simulink model "MVB3single"  (R2013b)
settings: Solver=FixedStepDiscrete  SolverMode=SingleTasking  StartTime=0  StopTime=5000  RelTol=1e-3
model workspace (MAT data in the model file):
  logicAddr = 2
settings Model: Creator=qiji  LastModifiedBy=qiji
settings DataIOCC: SignalLoggingSaveFormat=ModelDataLogs
settings OptimizationCC: BlockReduction=off  ConditionallyExecuteInputs=off  InlineParams=on
settings DebuggingCC: UnderspecifiedInitializationDetection=Simplified  MultiTaskDSMMsg=warning  MultiTaskCondExecSysMsg=none  SingleTaskRateTransMsg=error  SFUnusedDataAndEventsDiag=none
settings RTWCC: IncludeERTFirstTime=on
settings GRTTargetCC: CodeReplacementLibrary=None  CPPClassGenCompliant=on
settings ConfigurationSet: Description=SimMechanics 2G

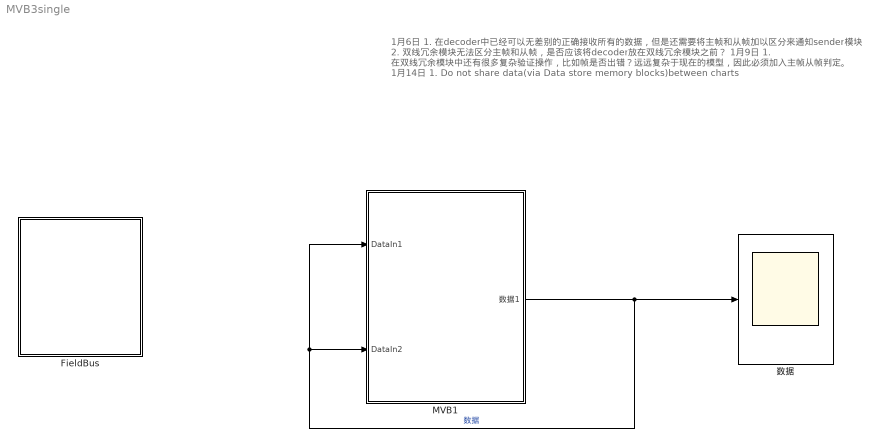
== system MVB3single ==
  note: 1月6日
      | 1. 在decoder中已经可以无差别的正确接收所有的数据，但是还需要将主帧和从帧加以区分来通知sender模块
      | 2. 双线冗余模块无法区分主帧和从帧，是否应该将decoder放在双线冗余模块之前？
      | 1月9日
      | 1. 在双线冗余模块中还有很多复杂验证操作，比如帧是否出错？远远复杂于现在的模型，因此必须加入主帧从帧判定。
      | 1月14日
      | 1. Do not share data(via Data store memory blocks)between charts
  FieldBus : Subsystem
  MVB1 : Subsystem
  数据 : Scope
  wires:
  MVB1/1(数据1) -> MVB1/2(DataIn2), MVB1/1(DataIn1), 数据/1  "数据"

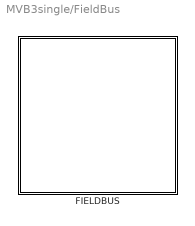
== system MVB3single/FieldBus ==
  FIELDBUS : Stateflow chart  TreatAsAtomicUnit=on

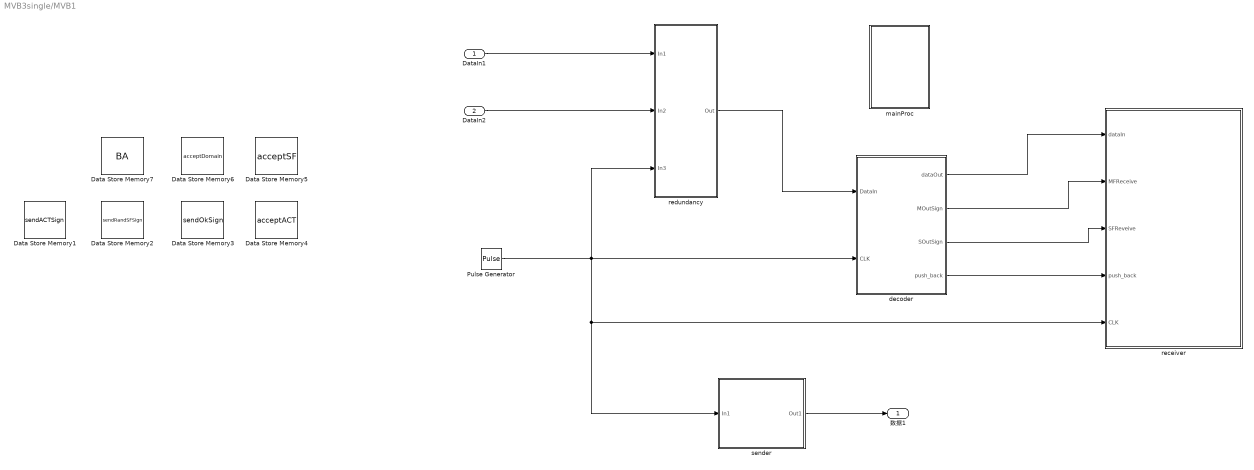
== system MVB3single/MVB1 ==
  DataIn1 : Inport
  DataIn2 : Inport  Port=2
  Data Store Memory1 : DataStoreMemory  DataStoreName=sendACTSign  ReadBeforeWriteMsg=warning  WriteAfterWriteMsg=warning  WriteAfterReadMsg=warning  OutDataTypeStr=boolean
  Data Store Memory2 : DataStoreMemory  DataStoreName=sendRandSFSign  ReadBeforeWriteMsg=warning  WriteAfterWriteMsg=warning  WriteAfterReadMsg=warning  OutDataTypeStr=boolean
  Data Store Memory3 : DataStoreMemory  DataStoreName=sendOkSign  ReadBeforeWriteMsg=warning  WriteAfterWriteMsg=warning  WriteAfterReadMsg=warning  OutDataTypeStr=boolean
  Data Store Memory4 : DataStoreMemory  DataStoreName=acceptACT  ReadBeforeWriteMsg=warning  WriteAfterWriteMsg=warning  WriteAfterReadMsg=warning  InitialValue=false  OutDataTypeStr=boolean
  Data Store Memory5 : DataStoreMemory  DataStoreName=acceptSF  ReadBeforeWriteMsg=warning  WriteAfterWriteMsg=warning  WriteAfterReadMsg=warning  InitialValue=false  OutDataTypeStr=boolean
  Data Store Memory6 : DataStoreMemory  DataStoreName=acceptDomain  ReadBeforeWriteMsg=warning  WriteAfterWriteMsg=warning  WriteAfterReadMsg=warning  InitialValue=false  OutDataTypeStr=boolean
  Data Store Memory7 : DataStoreMemory  DataStoreName=BA  ReadBeforeWriteMsg=warning  WriteAfterWriteMsg=warning  WriteAfterReadMsg=warning  InitialValue=true  OutDataTypeStr=boolean
  Pulse Generator : DiscretePulseGenerator  Amplitude=true
  decoder : Subsystem
  mainProc : Subsystem
  receiver : Subsystem
  redundancy : Subsystem
  sender : Subsystem
  数据1 : Outport
  wires:
  DataIn1/1 -> redundancy/1(In1)
  DataIn2/1 -> redundancy/2(In2)
  redundancy/1(Out) -> decoder/1(DataIn)
  sender/1(Out1) -> 数据1/1
  Pulse Generator/1 -> redundancy/3(In3), sender/1(In1), receiver/5(CLK), decoder/2(CLK)
  decoder/1(dataOut) -> receiver/1(dataIn)
  decoder/2(MOutSign) -> receiver/2("MFReceive ")
  decoder/3(SOutSign) -> receiver/3(SFReveive)
  decoder/4(push_back) -> receiver/4(push_back)

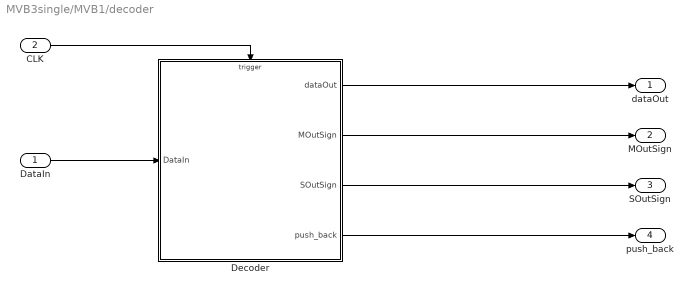
== system MVB3single/MVB1/decoder ==
  DataIn : Inport  OutDataTypeStr=uint32
  CLK : Inport  Port=2  OutDataTypeStr=boolean
  Decoder : Stateflow chart  TreatAsAtomicUnit=on
  dataOut : Outport
  MOutSign : Outport  Port=2
  SOutSign : Outport  Port=3
  push_back : Outport  Port=4
  wires:
  Decoder/3(SOutSign) -> SOutSign/1
  Decoder/2(MOutSign) -> MOutSign/1
  Decoder/4(push_back) -> push_back/1
  Decoder/1(dataOut) -> dataOut/1
  DataIn/1 -> Decoder/1(DataIn)
  CLK/1 -> Decoder/Trigger

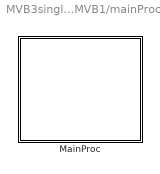
== system MVB3single/MVB1/mainProc ==
  MainProc : Stateflow chart  TreatAsAtomicUnit=on

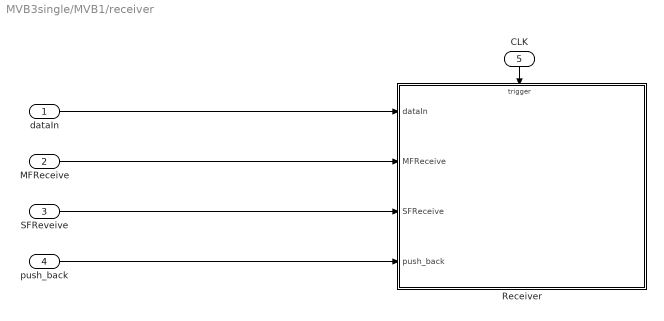
== system MVB3single/MVB1/receiver ==
  dataIn : Inport
  "MFReceive " : Inport  Port=2
  SFReveive : Inport  Port=3
  push_back : Inport  Port=4
  CLK : Inport  Port=5
  Receiver : Stateflow chart  TreatAsAtomicUnit=on
  wires:
  CLK/1 -> Receiver/Trigger
  "MFReceive "/1 -> Receiver/2(MFReceive)
  SFReveive/1 -> Receiver/3(SFReceive)
  dataIn/1 -> Receiver/1(dataIn)
  push_back/1 -> Receiver/4(push_back)

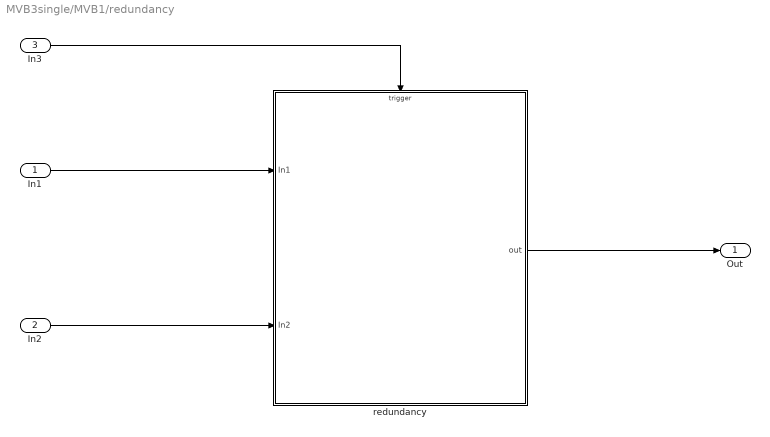
== system MVB3single/MVB1/redundancy ==
  In1 : Inport
  In2 : Inport  Port=2
  In3 : Inport  Port=3  OutDataTypeStr=boolean
  redundancy : Stateflow chart  TreatAsAtomicUnit=on
  Out : Outport
  wires:
  redundancy/1(out) -> Out/1
  In2/1 -> redundancy/2(In2)
  In1/1 -> redundancy/1(In1)
  In3/1 -> redundancy/Trigger

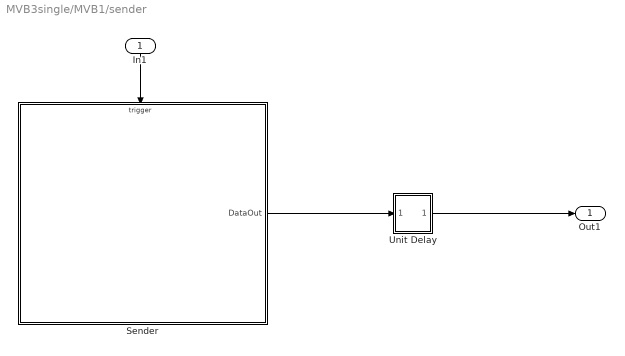
== system MVB3single/MVB1/sender ==
  In1 : Inport
  Sender : Stateflow chart  TreatAsAtomicUnit=on
  Unit Delay : Subsystem
  Out1 : Outport
  wires:
  Unit Delay/1(Out) -> Out1/1
  Sender/1(DataOut) -> Unit Delay/1(In1)
  In1/1 -> Sender/Trigger

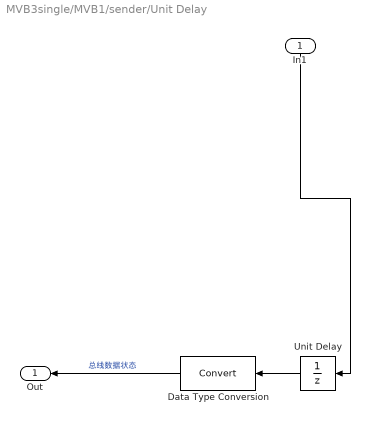
== system MVB3single/MVB1/sender/Unit Delay ==
  In1 : Inport
  Data Type Conversion : DataTypeConversion
  Unit Delay : UnitDelay  SampleTime=-1
  Out : Outport
  wires:
  In1/1 -> Unit Delay/1
  Unit Delay/1 -> Data Type Conversion/1
  Data Type Conversion/1 -> Out/1  "总线数据状态"

== stateflow chart MVB3single/FieldBus/FIELDBUS ==
  settings: executeAtInitialization=1  initializeOutput=1
  state IDLE
  state busy
  state space
  state turnFalse [function]
    (default) -> (junction 45) : {
        | trans1 = false;
        | trans2 = false;
        | trans3 = false;
        | }
  state r = pull(a, b, c) [function]
    (default) -> (junction 17)
    (junction 17) -> (junction 19) [order 1] : [a==true]{trans1=true; r=1;}
    (junction 17) -> (junction 21) [order 2]
    (junction 21) -> (junction 22) [order 1] : [b==true]{trans2=true; r=1;}
    (junction 21) -> (junction 24) [order 2]
    (junction 24) -> (junction 23) : [c==true]{trans3=true;r=1}
  state init [function]
    (default) -> (junction 40) : {
        | trans1 = false;
        | trans2 = false;
        | trans3 = false;
        | }
  IDLE -> busy : [pull(signal1, signal2, signal3)]
  (default) -> IDLE
  busy -> space : {t = clock_Counter}
  space -> IDLE : [clock_Counter - t > (50/prop)]{turnFalse()}
  data: r function_output double; a function_input double; b function_input double; c function_input double; t local uint32; clock_Counter local uint32; trans1 local double; trans2 local double; trans3 local double; signal1 local double; signal2 local double; signal3 local double; prop local double

== stateflow chart MVB3single/MVB1/receiver/Receiver ==
  settings: sampleTime=4.1666666667e-8  initializeOutput=1
  state receiveSF [parallel]
    settings: executionOrder=2
    note: acceptSF, acceptACT, acceptDomain在发送完主帧以后，根据主帧的类型进行相应的置位
        | 收到fcode为8的从帧之后，说明目标设备已经返回了OK，这时应该将BA设为1
    state wait
      en:
      initBuffer();
    state wait4SFEnd
    state judge4SF
    state wait4SF
    state wait4ACT
    state wait4Domain
    state STrans
    (default) -> receiveSF.wait
    (junction 96) -> receiveSF.wait : {
        | BufferIndex = 0;
        | }
    receiveSF.wait -> wait4SFEnd : [SFReceive == true]
    wait4SFEnd -> judge4SF : [SFReceive == false]
    judge4SF -> (junction 96) [order 4]
    STrans -> (junction 96) : [SFReceive == false]
    judge4SF -> wait4Domain [order 3] : [acceptDomain == true]
    judge4SF -> wait4SF [order 1] : [acceptSF == true]
    judge4SF -> wait4ACT [order 2] : [acceptACT == true]
    wait4SF -> STrans : {
        | acceptSF = false;
        | }
    wait4ACT -> STrans : [getbit(buffer[1], 6)]
        | {
        | acceptACT = false;
        | }
    wait4Domain -> STrans : [getbit(buffer[1], 8) == 1]
        | {
        | acceptDomain = false;
        | BA = false;
        | }
  state receiveMF [parallel]
    settings: executionOrder=1
    state wait
      en:
      initBuffer();
    state wait4MFEnd
    state judgeAddr
    state MFReceive
    state MFcode0
    state MFcode8
    state MFcode15
    state MTrans
    (default) -> receiveMF.wait
    judgeAddr -> receiveMF.wait [order 2]
    MTrans -> receiveMF.wait : [sendRandSFSign == false && sendOkSign == false && sendACTSign == false]
    receiveMF.wait -> wait4MFEnd : [MFReceive==true]
    wait4MFEnd -> judgeAddr : [MFReceive == false]
        | {fcodeIn = uint8(getFCode(buffer));
        | addrIn = uint16(getAddr(buffer));
        | }
    judgeAddr -> MFReceive [order 1] : [addrIn == LogicAddr]
    MFReceive -> MFcode0 [order 2] : [fcodeIn == 0]
    MFReceive -> MFcode8 [order 3] : [fcodeIn == 8]
    MFReceive -> MFcode15 [order 1] : [fcodeIn == 15 ]
    MFcode0 -> MTrans : {sendRandSFSign = true}
    MFcode8 -> MTrans : {sendACTSign = true}
    MFcode15 -> MTrans : {sendOkSign = true}
  state initBuffer [function]
    (default) -> (junction 159) : /* init Buffer */
        | {BufferIndex=0;}
    (junction 158) -> (junction 156) [order 1] : [index<16]
    (junction 156) -> (junction 157) : {buffer[index] = 0;}
    (junction 159) -> (junction 158) : {index=0;}
    (junction 157) -> (junction 158) : {index++;}
    (junction 158) -> (junction 155) [order 2]
  state Buffer [parallel]
    settings: executionOrder=3
    state wait
    state push_back
      en:
      buffer[BufferIndex]=dataIn;
      BufferIndex = BufferIndex+1;
    (default) -> Buffer.wait : {
        | BufferIndex=0;
        | }
    Buffer.wait -> push_back : [push_back==1]
    push_back -> Buffer.wait
  note: 期待目标设备返回OK
  data: index local double; data function_input uint32; num function_input uint32; r function_output uint32; data function_input uint16 size=16; r function_output uint16; bit1 temporary uint16; bit2 temporary uint16; bit3 temporary uint16; bit0 temporary uint16; data function_input uint32; r function_output uint32; r function_output uint32; data function_input uint32; data function_input uint16 size=16; r function_output uint16; dataIn input uint32; MFReceive input boolean; SFReceive input boolean; fcodeIn local uint8; addrIn local uint16; sendRandSFSign data_store_memory; sendOkSign data_store_memory; sendACTSign data_store_memory; acceptSF data_store_memory; acceptDomain data_store_memory; acceptACT data_store_memory; BA data_store_memory; BufferIndex local double; buffer local uint16 size=16 =[0,0,0,0,0,0,0,0,0,0,0,0,0,0,0,0]; push_back input boolean; LogicAddr constant uint8 =1
  events: CLK input RISING_EDGE_EVENT
  function r = getbit(data, num):
    | function r = getbit(data, num)
    | r = bitget(uint32(data), num);
  function r = getFCode(data):
    | function r = getFCode(data)
    | bit0 = bitget(data(2), 9);
    | bit1 = bitget(data(2), 10);
    | bit2 = bitget(data(2), 11);
    | bit3 = bitget(data(2), 12);
    | r = bit0+bit1*2+bit2*4+bit3*8;
  function r = ManchesterEncoding(data):
    | function r = ManchesterEncoding(data)
    | r = data;
    | for i = 1:16
    |     x = bitget(data, i);
    |     if x == 0
    |         r = bitset(r, i*2-1, 1);
    |         r = bitset(r, i*2, 0);
    |     else
    |         r = bitset(r, i*2-1, 0);
    |         r = bitset(r, i*2, 1);
    |     end
    | end
  function r = ManchesterDecoding(data):
    | function r = ManchesterDecoding(data)
    | r = uint32(0);
    | for i = (1:2:32)
    |     x0 = bitget(data, i);
    |     x1 = bitget(data, i+1);
    |     if x0==0 && x1==1
    |         r = bitset(r, (i+1)/2, 1);
    |     else
    |         r = bitset(r, (i+1)/2, 0);
    |     end
    | end
  function r = getAddr(data):
    | function r = getAddr(data)
    | %取出buffer(2)后8位
    | high8 = bitshift(bitshift(uint16(data(2)), 8), -4);
    | % 取出buffer(3)前4位
    | low4 = bitshift(uint16(data(3)), -12);
    | r = high8 + low4;

== stateflow chart MVB3single/MVB1/decoder/Decoder ==
  settings: initializeOutput=1
  state judge_data [parallel]
    settings: executionOrder=2
    state MF
      en:
      MOutSign= true;
    state wait4Data
      en:
      initBuffer();
    state judgeData
    state end
      en:
      MOutSign=false;
      SOutSign=false;
    state SF
      en:
      SOutSign=true;
    judgeData -> MF [order 1] : [judge(buffer)==1]
    MF -> end
    wait4Data -> judgeData : receive_complete
    (default) -> wait4Data
    judgeData -> wait4Data [order 3] : [judge(buffer)==0]
    judgeData -> SF [order 2] : [judge(buffer)==2]
    end -> wait4Data
    SF -> end
  state initBuffer [function]
    (default) -> (junction 129) : /* init Buffer */
        | {index=0;}
    (junction 119) -> (junction 123) [order 1] : [i<16]
    (junction 123) -> (junction 125) : {buffer[i] = 0;}
    (junction 129) -> (junction 119) : {i=0;}
    (junction 125) -> (junction 119) : {i++;}
    (junction 119) -> (junction 118) [order 2]
  note: 0010//1100/0111/0001
      | 0101//0000/0000/0000
      | 0001//1010/1000/1110
      | 0000/0000/0011//0011
  state receiver [parallel]
    settings: executionOrder=1
    state decodeSF
      decodeSF -> decodeSF [order 1] : CLK
          | {
          | ans = bitoperate.shiftbit(ans, 1) + DataIn;
          | count++;
          | }
    note: 首先接受所有的数据，当接受完毕以后，再通知另外一个子系统判断
        | 从帧和主帧，并对dataout赋值。
    state judge
      en:
      ans = 0;
      ex:
      push_back = 1 - push_back;
    state start
    decodeSF -> judge [order 1] : [count==32]
        | {
        | dataOut = ManchesterDecoding(ans);
        | count=0;
        | buffer[index] = dataOut;
        | push_back = 1 - push_back;
        | }
    start -> decodeSF : [DataIn == 1]
        | {
        | count = 2;
        | ans=1;
        | }
    judge -> decodeSF [order 1] : [!judgeEnd(buffer[index])]
        | {index++;}
    judge -> start [order 2] : {
        | send(receive_complete, judge_data);
        | dataOut = 0;
        | }
    (default) -> start : {
        | push_back =0;
        | }
  state bitoperate [group]
  data: r function_output double; dataBuffer function_input uint16 size=16; i temporary double; r function_output boolean; data function_input uint16; num function_input uint32; r function_output uint32; data function_input uint32; num function_input uint32; r function_output uint32; r function_output uint32; data function_input uint32; DataIn input uint32; dataOut output uint32; count local uint32; MOutSign output boolean; SOutSign output boolean; ans local uint32; buffer local uint16 size=16; index local double; push_back output boolean
  events: CLK input RISING_EDGE_EVENT; receive_complete local FUNCTION_CALL_EVENT
  function r = judge(dataBuffer):
    | function r = judge(dataBuffer)
    | low12 = bitshift(dataBuffer(1), 4);
    | high4 = bitshift(dataBuffer(2), -12);
    | start = low12 + high4;
    | r = 0;
    | if start == 50965
    |     r = 1;
    | elseif start == 43235
    |     r = 2;
    | end
  function r = judgeEnd(data):
    | function r = judgeEnd(data)
    | bit1 = bitget(data, 1);
    | bit2 = bitget(data, 2);
    | bit3 = bitget(data, 3);
    | bit4 = bitget(data, 4);
    | if bit1==1 && bit2==1 && bit3==0 && bit4==0
    |     r = true;
    | else
    |     r = false;
    | end
  function r = getbit(num):
    | function r = getbit(num)
    | r = bitget(num, 32);
  function r = shiftbit(data, num):
    | function r = shiftbit(data, num)
    | r = bitshift(data, num);
    | %for i=1:cnt
    | %   r = bitset(r, i, 0);
    | %end
  function r = ManchesterDecoding(data):
    | function r = ManchesterDecoding(data)
    | r = uint32(0);
    | for i = (1:2:32)
    |     x0 = bitget(data, i);
    |     x1 = bitget(data, i+1);
    |     if x0==0 && x1==1
    |         r = bitset(r, (i+1)/2, 1);
    |     else
    |         r = bitset(r, (i+1)/2, 0);
    |     end
    | end

== stateflow chart MVB3single/MVB1/mainProc/MainProc ==
  settings: executeAtInitialization=1  initializeOutput=1
  state mainproc [parallel]
    settings: executionOrder=1
    state StandbyEquip
    state MainEquip
    state wait4ACT
    note: 等待其他设备返回ACT
    note: 等待其他设备返回OK，receiver在接收到OK以后立马放弃主权
    state TempEquip
    (default) -> StandbyEquip
    TempEquip -> StandbyEquip : [BA == false]
    StandbyEquip -> MainEquip : [BA == true && ACT == true]
    MainEquip -> wait4ACT : [acceptACT == true]
    wait4ACT -> TempEquip : [acceptDomain == true]
  data: BA data_store_memory; ACT local boolean =true; acceptACT data_store_memory; acceptDomain data_store_memory

== stateflow chart MVB3single/MVB1/sender/Sender ==
  settings: initializeOutput=1
  state init [function]
    note: F_code=0
        | addr=2
        | 0010//1100/0111/0001
        | 0101//0000/0000/0000
        | 0010//1010/1000/1110
        | 0000/0000/0011//0011
        | F_code=8
        | addr=2
        | 0010//1100/0111/0001
        | 0101//1000/0000/0000
        | 0010//1010/1000/1110
        | 0000/0000/0011//0011
        | F_code=0
        | addr=2
        | 0010//1100/0111/0001
        | 0101//1111/0000/0000
        | 0010//1010/1000/1110
        | 0000/0000/0011//0011
    note: 请求随机从帧
        | 请求随机从帧
        | 请求2号的信息
        | 请求转移到2号
    note: SFT(1)代表随机的从帧
        | SFT(2)代表回复接受主权
        | SFT(3)代表回复设备ACT和BA
    (default) -> (junction 100) : {
        | BA = true;
        | MFIndex = 0;
        | SendSignal = false;
        |
        | MFT(1) = 5;
        | MFT(2) = 11377;
        | MFT(3) = 20480;
        | MFT(4) = 6798;
        | MFT(5) = 51;
        |
        | MFT(17) = 5;
        | MFT(18) = 11377;
        | MFT(19) = 20480;
        | MFT(20) = 6798;
        | MFT(21) = 51;
        |
        | MFT(33) = 5;
        | MFT(34) = 11377;
        | MFT(35) = 22528;
        | MFT(36) = 10894;
        | MFT(37) = 51;
        |
        | MFT(49) = 5
        | MFT(50) = 11377;
        | MFT(51) = 24320;
        | MFT(52) = 10894;
        | MFT(53) = 51;
        |
        |
        | SFT(1) = 4;
        | SFT(2) = 10894;
        | SFT(3) = 12428;
        | SFT(4) = 19;
        | SFT(17) = 4;
        | SFT(18) = 10894;
        | SFT(19) = 12832;
        | SFT(20) = 3;
        | SFT(33) = 4;
        | SFT(34) = 10894;
        | SFT(35) = 14464;
        | SFT(36) = 3;
        | clock_3M_shang = false;
        | sendRandSFSign = false;
        | sendACTSign = false;
        | sendRandSFSign = false;
        | }
  state SFSender [parallel]
    settings: executionOrder=2
    note: send**Signd的置位在接收到了请求数据的主帧后置位
    state sender [parallel]
      settings: executionOrder=1
      state wait
      state sendRandomSF
      state sendOK
      state sendInfo
      state transmission
      (default) -> SFSender.sender.wait
      SFSender.sender.wait -> sendRandomSF [order 1] : [sendRandSFSign == true]
      SFSender.sender.wait -> sendInfo [order 3] : [sendACTSign == true]
      SFSender.sender.wait -> sendOK [order 2] : [sendOkSign == true]
      sendRandomSF -> SFSender.sender.transmission : {SFIndex = 0;
          | sendRandSFSign = false;}
      sendOK -> SFSender.sender.transmission : {SFIndex = 2;
          | sendOkSign = false;
          | init();
          | BA = true;
          | }
      sendInfo -> SFSender.sender.transmission : {SFIndex = 1;
          | sendACTSign = false;}
      SFSender.sender.transmission -> SFSender.sender : SFTransDone
          | {DataOut = uint32(0);
          | }
    state sendHolder [parallel]
      settings: executionOrder=2
      state judge
      state full
        SFSender.sendHolder.full -> SFSender.sendHolder.full [order 1] : CLK
            | {
            | DataOut = bitoperate.getbit(input);
            | input = bitoperate.shiftbit(input, uint32(1));
            | count = count + 1;
            | }
      state empty
      SFSender.sendHolder.judge -> SFSender.sendHolder.empty [order 2] : {
          | SFCurrentIndex = 2;
          | send(SFTransDone, sender);
          | }
      SFSender.sendHolder.full -> SFSender.sendHolder.judge [order 1] : [count == 32]
          | {
          | SFCurrentIndex = SFCurrentIndex + 1;
          | }
      SFSender.sendHolder.judge -> SFSender.sendHolder.full [order 1] : [SFCurrentIndex <= SFT(SFIndex*16 + 1)]
          | {
          | input = ManchesterEncoding(uint32(SFT(SFIndex*16+SFCurrentIndex)));
          | count = 0;
          | }
      (default) -> SFSender.sendHolder.empty : {
          | SFCurrentIndex = 2;
          | }
      SFSender.sendHolder.empty -> SFSender.sendHolder.full : enter(sender.transmission)
          | {
          | input = ManchesterEncoding(uint32(SFT(SFIndex*16+SFCurrentIndex)));
          | DataOut = uint32(0);
          | count = 0;
          | }
  state MFSender [parallel]
    settings: executionOrder=1
    state sender [parallel]
      settings: executionOrder=1
      state transmission
        entry:
        [acceptSF, acceptACT, acceptDomain] =setAcceptSignal(MFT(MFIndex*16+3));
      state sleep
      state wait
      (default) -> sleep : {
          | init();
          | flag= true;
          | }
      MFSender.sender.transmission -> sleep : MFTransDone
          | {
          | DataOut = uint32(0);
          | MFIndex = MFIndex + 1;
          | MFIndex  = reset(MFIndex);
          | }
      sleep -> MFSender.sender.wait : every(150, CLK)
          | [BA==true]
      MFSender.sender.wait -> MFSender.sender.transmission
    state sendHolder [parallel]
      settings: executionOrder=2
      state judge
      state full
        MFSender.sendHolder.full -> MFSender.sendHolder.full [order 1] : CLK
            | {
            | DataOut = bitoperate.getbit(input);
            | input = bitoperate.shiftbit(input, uint32(1));
            | count = count + 1;
            | }
      state empty
      MFSender.sendHolder.judge -> MFSender.sendHolder.empty [order 2] : {
          | MFCurrentIndex = 2;
          | send(MFTransDone, sender);
          | }
      MFSender.sendHolder.full -> MFSender.sendHolder.judge [order 1] : [count == 32]
          | {
          | MFCurrentIndex = MFCurrentIndex + 1;
          | }
      MFSender.sendHolder.judge -> MFSender.sendHolder.full [order 1] : [MFCurrentIndex <= MFT(MFIndex*16 + 1)]
          | {
          | input =ManchesterEncoding(uint32(MFT(MFIndex*16+MFCurrentIndex)));
          | count = 0;
          | }
      (default) -> MFSender.sendHolder.empty : {
          | MFCurrentIndex = 2;
          | }
      MFSender.sendHolder.empty -> MFSender.sendHolder.full : enter(sender.transmission)
          | {
          | input = ManchesterEncoding(uint32(MFT(MFIndex*16+MFCurrentIndex)));
          | DataOut = uint32(0);
          | count = 0;
          | }
  note: MFT(1) = 5;
      | MFT(2) = 11377;
      | MFT(3) = 20480;
      | MFT(4) = 10894;
      | MFT(5) = 51;
      |
      | MFT(17) = 5;
      | MFT(18) = 11377;
      | MFT(19) = 20480;
      | MFT(20) = 10894;
      | MFT(21) = 51;
      |
      | MFT(33) = 5;
      | MFT(34) = 11377;
      | MFT(35) = 22528;
      | MFT(36) = 10894;
      | MFT(37) = 51;
      |
      | MFT(49) = 5
      | MFT(50) = 11377;
      | MFT(52) = 24320;
      | MFT(53) = 10894;
      | MFT(54) = 51;
  state bitoperate [group]
  data: SFCurrentIndex local double; count local double; input local uint32; SFIndex local double; data function_input uint16; SF function_output boolean; bit1 temporary uint16; bit2 temporary uint16; bit3 temporary uint16; bit0 temporary uint16; ACT function_output boolean; Domain function_output boolean; flag local boolean; MFCurrentIndex local double; count local double; input local uint32; data function_input uint32; r function_output uint32; r function_output uint32; data function_input uint32; num function_input uint32; r function_output uint32; data function_input uint32; num function_input uint32; r function_output uint32; i function_input double; r function_output double; DataOut output uint32; MFIndex local; MFT local uint16 size=100; sendOkSign data_store_memory; sendRandSFSign data_store_memory; sendACTSign data_store_memory; acceptSF data_store_memory; BA data_store_memory; acceptACT data_store_memory; acceptDomain data_store_memory; SFT local uint16 size=100
  events: SFTransDone local FUNCTION_CALL_EVENT; MFTransDone local FUNCTION_CALL_EVENT; CLK input RISING_EDGE_EVENT
  function [SF, ACT, Domain] = setAcceptSignal(data):
    | function [SF, ACT, Domain] = setAcceptSignal(data)
    | bit0 = uint16(bitget(data, 9));
    | bit1 = uint16(bitget(data, 10));
    | bit2 = uint16(bitget(data, 11));
    | bit3 = uint16(bitget(data, 12));
    | fcode = bit0+bit1*2+bit2*4+bit3*8;
    | SF=false;
    | ACT=false;
    | Domain=false;
    | if fcode==0
    |     SF=true;
    | elseif fcode==8
    |     ACT=true;
    | elseif fcode==15
    |     Domain=true;
    | end
  function r = ManchesterEncoding(data):
    | function r = ManchesterEncoding(data)
    | r = data;
    | for i = 1:16
    |     x = bitget(data, i);
    |     if x == 0
    |         r = bitset(r, i*2-1, 1);
    |         r = bitset(r, i*2, 0);
    |     else
    |         r = bitset(r, i*2-1, 0);
    |         r = bitset(r, i*2, 1);
    |     end
    | end
  function r = ManchesterDecoding(data):
    | function r = ManchesterDecoding(data)
    | r = uint32(0);
    | for i = (1:2:32)
    |     x0 = bitget(data, i);
    |     x1 = bitget(data, i+1);
    |     if x0==0 && x1==1
    |         r = bitset(r, (i+1)/2, 1);
    |     else
    |         r = bitset(r, (i+1)/2, 0);
    |     end
    | end
  function r = getbit(num):
    | function r = getbit(num)
    | r = bitget(num, 32);
  function r = shiftbit(data, num):
    | function r = shiftbit(data, num)
    | r = bitshift(data, num);
    | %for i=1:cnt
    | %   r = bitset(r, i, 0);
    | %end
  function r = reset(i):
    | function r = reset(i)
    | if i==2
    |     r = 0;
    | else
    |     r=i;
    | end

== stateflow chart MVB3single/MVB1/redundancy/redundancy ==
  settings: executeAtInitialization=1  initializeOutput=1
  state sign_maker [parallel]
    settings: executionOrder=1
    state sign1 [parallel]
      settings: executionOrder=1
      state trans
        sign_maker.sign1.trans -> sign_maker.sign1.trans [order 1] : CLK
            | {
            | buffer = bitoperate.shiftbit(buffer, 1) + In1;
            | count++;
            | }
      state none
        en:
        count=2;
        buffer=1;
      state judge
      (default) -> sign_maker.sign1.none : {count=0;buffer=0;}
      sign_maker.sign1.none -> sign_maker.sign1.trans : [In1==1]{sign1 = true;}
      sign_maker.sign1.judge -> sign_maker.sign1.trans [order 2] : {buffer=0;count=0;}
      sign_maker.sign1.judge -> sign_maker.sign1.none [order 1] : [judgeEnd(buffer)]
          | {sign1 = false;}
      sign_maker.sign1.trans -> sign_maker.sign1.judge [order 1] : [count==32]
          | {buffer=ManchesterDecoding(buffer);
          | }
    state sign2 [parallel]
      settings: executionOrder=2
      state trans
        sign_maker.sign2.trans -> sign_maker.sign2.trans [order 1] : CLK
            | {
            | buffer = bitoperate.shiftbit(buffer, 1) + In2;
            | count++;
            | }
      state none
        en:
        count=2;
        buffer=1;
      state judge
      (default) -> sign_maker.sign2.none : {count=0;buffer=0;}
      sign_maker.sign2.none -> sign_maker.sign2.trans : [In2==1]{sign2 = true;}
      sign_maker.sign2.judge -> sign_maker.sign2.trans [order 2] : {buffer=0;count=0;}
      sign_maker.sign2.judge -> sign_maker.sign2.none [order 1] : [judgeEnd(buffer)]
          | {sign2 = false;}
      sign_maker.sign2.trans -> sign_maker.sign2.judge [order 1] : [count==32]
          | {buffer=ManchesterDecoding(buffer);
          | }
  state bitoperate [group]
  note: 从上一个接收事件后总线寂静1.4ms则产生一总线寂静的通知
  state Timer1 [parallel]
    settings: executionOrder=2
    state Timer
    state start
    state TimeOut
      entry:
      trust = false;
    start -> Timer : [judge(sign1, sign2, trust) == false]
    (default) -> start
    Timer -> start [order 1] : [judge(sign1, sign2,  trust) == true]
    TimeOut -> start
    Timer -> TimeOut [order 2] : [after(140, CLK) && judge(sign1, sign2,  trust) == false]
  note: 上一个主帧接收后1.3ms没有收到主帧产生一个主帧超时的通知。
  note: 收到主帧后42.7us没有收到从帧产生从帧超时的通知。
  note: 信任线未收到数据，而观察线收到数据时切换
  state observer [parallel]
    settings: executionOrder=3
    state A
      entry:
      trust = true;
    state B
      entry:
      trust = false;
    observer.A -> observer.B : [judge(sign1, sign2, trust) == false]
    (default) -> observer.A
    observer.B -> observer.A : [judge(sign1, sign2, trust) == false]
  state trans [parallel]
    settings: executionOrder=4
    state A
      during:
      out = In1;
    state B
      during:
      out = In2;
    trans.A -> trans.B : [trust == false]{out = In2;}
    (default) -> trans.A
    trans.B -> trans.A : [trust == true]{out = In1;}
  data: r function_output boolean; data function_input uint16; buffer local uint32; count local uint32; buffer local uint32; count local uint32; r function_output uint32; data function_input uint32; num function_input uint32; r function_output uint32; data function_input uint32; num function_input uint32; r function_output uint32; r function_output boolean; dataIn1 function_input uint32; dataIn2 function_input uint32; t function_input boolean; r function_output boolean; dataIn1 function_input boolean; dataIn2 function_input boolean; t function_input boolean; In1 input uint32; In2 input uint32; out output uint32; trust local boolean =true; sign1 local boolean; sign2 local boolean
  events: CLK input RISING_EDGE_EVENT
  function r = judgeEnd(data):
    | function r = judgeEnd(data)
    | bit1 = bitget(data, 1);
    | bit2 = bitget(data, 2);
    | bit3 = bitget(data, 3);
    | bit4 = bitget(data, 4);
    | if bit1==1 && bit2==1 && bit3==0 && bit4==0
    |     r = true;
    | else
    |     r = false;
    | end
  function r = ManchesterDecoding(data):
    | function r = ManchesterDecoding(data)
    | r = uint32(0);
    | for i = (1:2:32)
    |     x0 = bitget(data, i);
    |     x1 = bitget(data, i+1);
    |     if x0==0 && x1==1
    |         r = bitset(r, (i+1)/2, 1);
    |     else
    |         r = bitset(r, (i+1)/2, 0);
    |     end
    | end
  function r = getbit(num):
    | function r = getbit(num)
    | r = bitget(num, 32);
  function r = shiftbit(data, num):
    | function r = shiftbit(data, num)
    | r = bitshift(data, num);
    | %for i=1:cnt
    | %   r = bitset(r, i, 0);
    | %end
  function r = judge(dataIn1, dataIn2, t):
    | function r = judge(dataIn1, dataIn2, t)
    | r = true;
    | if t == true
    |     if dataIn1==false
    |         r = false;
    |     end
    | else
    |     if dataIn2==false
    |         r = false;
    |     end
    | end
  function r = judge( dataIn1, dataIn2, t):
    | function r = judge( dataIn1, dataIn2, t)
    | r = true;
    | % 如果数据线1没有收到数据而数据线2收到了
    | if t == true
    |     if dataIn1==false && dataIn2==true
    |         r = false;
    |     end
    | else
    |     if dataIn2==false && dataIn1==true
    |         r = false;
    |     end
    | end
